simulink model "generalized_ess_test"  (R2021b)
settings: Solver=VariableStepAuto  StartTime=0.0  StopTime=3600  RelTol=1e-3
InitFcn:
  | %energy storage system
  | ess.Vdc_nom = 100;
  | ess.Vdc_0 = 100; %V
  | ess.Vdc_del = 50;
  | %ess.storageType = "bat"; %"sc" for supercapacitor, "bat" for battery
  | ess.storageType = "sc"; %"sc" for supercapacitor, "bat" for battery
  | 
  | ess.Ecap = 10; %total energy storage capacity, Wh
  | ess.isActive = 1;
  | ess.Cdc = 100e-6;
  | ess.kp_v = 0;
  | ess.ki_v = 0;
  | 
  | 
  | %determines the model parameters based on storage type, capacity, and
  | %nominal voltage
  | if ess.storageType == "bat"
  |     ess = ess_passive_bat_config(ess);
  | else %for now assume if not bat, do sc
  |     ess = ess_passive_sc_config(ess);
  | end
settings Model: Creator=jacksder  LastModifiedBy=Derek

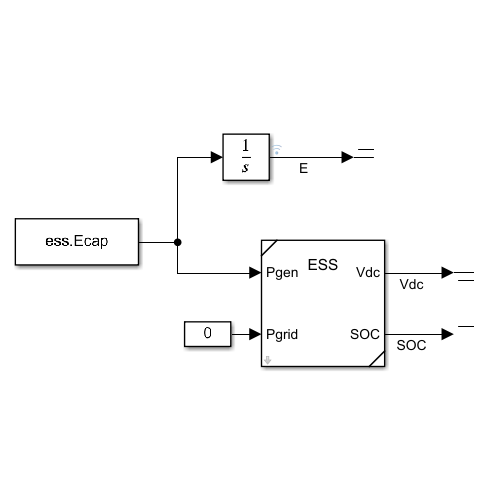
[thumbnail: Simulink's stored preview of the top-level diagram]
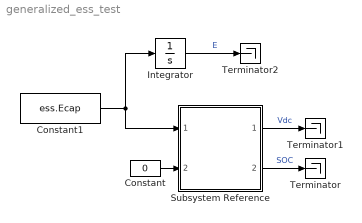
== system generalized_ess_test ==
  Constant : Constant  Value=0
  Constant1 : Constant  Value=ess.Ecap
  Integrator : Integrator
  Subsystem Reference : Subsystem  ReferencedSubsystem=ESS  ess=ess
  Terminator : Terminator
  Terminator1 : Terminator
  Terminator2 : Terminator
  wires:
  Constant/1 -> Subsystem Reference/2
  Constant1/1 -> Subsystem Reference/1, Integrator/1
  Subsystem Reference/2 -> Terminator/1  "SOC"
  Subsystem Reference/1 -> Terminator1/1  "Vdc"
  Integrator/1 -> Terminator2/1  "E"
